simulink model "tst_bus_outputasbus_hierarchy"  (Simulink 8.0)
settings: Solver=ode45  StartTime=0.0  StopTime=10.0  RelTol=1e-3
settings Model: Creator=Marci  LastModifiedBy=Marci

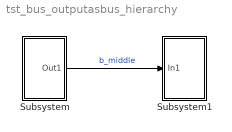
== system tst_bus_outputasbus_hierarchy ==
  Subsystem : Subsystem
  Subsystem1 : Subsystem
  wires:
  Subsystem/1(Out1) -> Subsystem1/1(In1)  "b_middle"

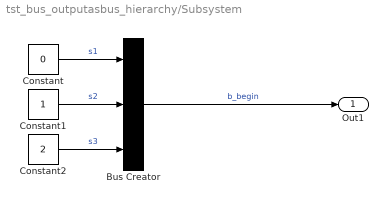
== system tst_bus_outputasbus_hierarchy/Subsystem ==
  Bus Creator : BusCreator  Inputs=3
  Constant : Constant  Value=0
  Constant1 : Constant
  Constant2 : Constant  Value=2
  Out1 : Outport
  wires:
  Constant2/1 -> Bus Creator/3  "s3"
  Constant1/1 -> Bus Creator/2  "s2"
  Constant/1 -> Bus Creator/1  "s1"
  Bus Creator/1 -> Out1/1  "b_begin"

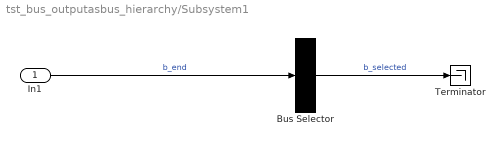
== system tst_bus_outputasbus_hierarchy/Subsystem1 ==
  In1 : Inport
  Bus Selector : BusSelector  OutputSignals=s2,s3  OutputAsBus=on
  Terminator : Terminator
  wires:
  In1/1 -> Bus Selector/1  "b_end"
  Bus Selector/1 -> Terminator/1  "b_selected"
